simulink model "full_R2016b"  (R2017a)
settings: Solver=VariableStepAuto  StartTime=0.0  StopTime=10.0  RelTol=1e-3
libraries: aerolibconvert2 x2, aerolibgravity2 x2
settings Model: Creator=decla  LastModifiedBy=decla
settings DataIOCC: ReturnWorkspaceOutputs=on
settings SFSimCC: SimUseLocalCustomCode=on
settings RTWCC: RTWUseLocalCustomCode=on

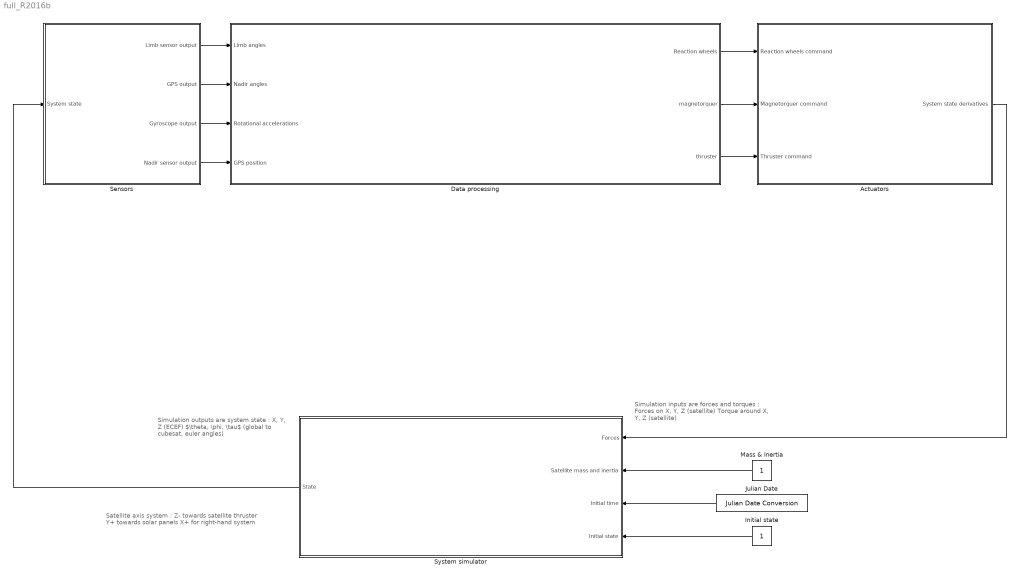
== system full_R2016b ==
  note: Simulation outputs are system state :
      | X, Y, Z (ECEF)
      | $\theta, \phi, \tau$ (global to cubesat, euler angles)
  note: Simulation inputs are forces and torques :
      | Forces on X, Y, Z (satellite)
      | Torque around X, Y, Z (satellite)
  note: Satellite axis system :
      | Z- towards satellite thruster
      | Y+ towards solar panels
      | X+ for right-hand system
  Actuators : Subsystem
  Data processing : Subsystem
  Initial state : Constant
  Julian Date : aerolibconvert2/Julian Date Conversion  year=2004  month=October  day=10  hour=12  min=21  sec=0  modflag=off  deltaT=None  errorflag=Error
      settings: SourceProductBaseCode=AE
  Mass & Inertia : Constant
  Sensors : Subsystem
  System simulator : Subsystem
  wires:
  Data processing/3(thruster) -> Actuators/3(Thruster command)
  Actuators/1(System state derivatives) -> System simulator/1(Forces)
  System simulator/1(State) -> Sensors/1(System state)
  Sensors/4(Nadir sensor output) -> Data processing/4(GPS position)
  Sensors/3(Gyroscope output) -> Data processing/3(Rotational accelerations)
  Sensors/2(GPS output) -> Data processing/2(Nadir angles)
  Sensors/1(Limb sensor output) -> Data processing/1(Limb angles)
  Data processing/2(magnetorquer) -> Actuators/2(Magnetorquer command)
  Data processing/1(Reaction wheels) -> Actuators/1(Reaction wheels command)
  Mass & Inertia/1 -> System simulator/2(Satellite mass and inertia)
  Julian Date/1 -> System simulator/3(Initial time)
  Initial state/1 -> System simulator/4(Initial state)

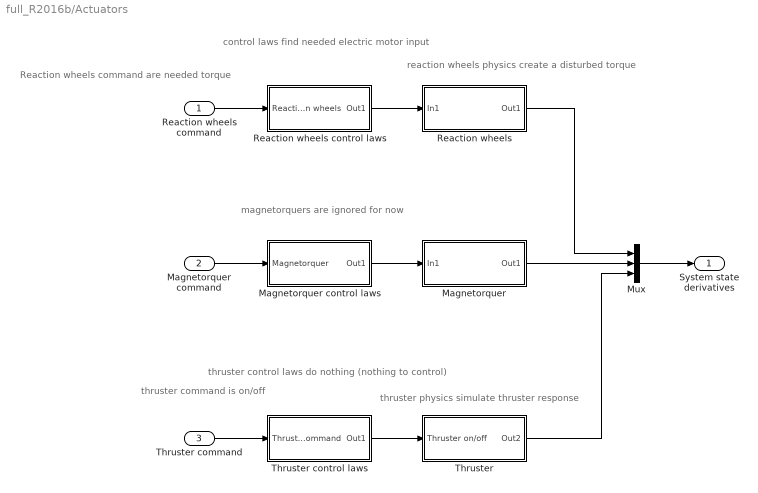
== system full_R2016b/Actuators ==
  note: magnetorquers are ignored for now
  note: thruster control laws do nothing (nothing to control)
  note: thruster physics simulate thruster response
  note: thruster command is on/off
  note: reaction wheels physics create a disturbed torque
  note: control laws find needed electric motor input
  note: Reaction wheels command are needed torque
  Reaction wheels command : Inport
  Magnetorquer command : Inport  Port=2
  Thruster command : Inport  Port=3
  Magnetorquer : Subsystem
  Magnetorquer control laws : Subsystem
  Mux : Mux  Inputs=3
  Reaction wheels : Subsystem
  Reaction wheels control laws : Subsystem
  Thruster : Subsystem
  Thruster control laws : Subsystem
  System state derivatives : Outport
  wires:
  Reaction wheels command/1 -> Reaction wheels control laws/1(Reaction wheels)
  Magnetorquer command/1 -> Magnetorquer control laws/1(Magnetorquer)
  Thruster command/1 -> Thruster control laws/1(Thruster command)
  Thruster control laws/1(Out1) -> Thruster/1(Thruster on/off)
  Magnetorquer control laws/1(Out1) -> Magnetorquer/1(In1)
  Reaction wheels control laws/1(Out1) -> Reaction wheels/1(In1)
  Thruster/1(Out2) -> Mux/3
  Magnetorquer/1(Out1) -> Mux/2
  Reaction wheels/1(Out1) -> Mux/1
  Mux/1 -> System state derivatives/1

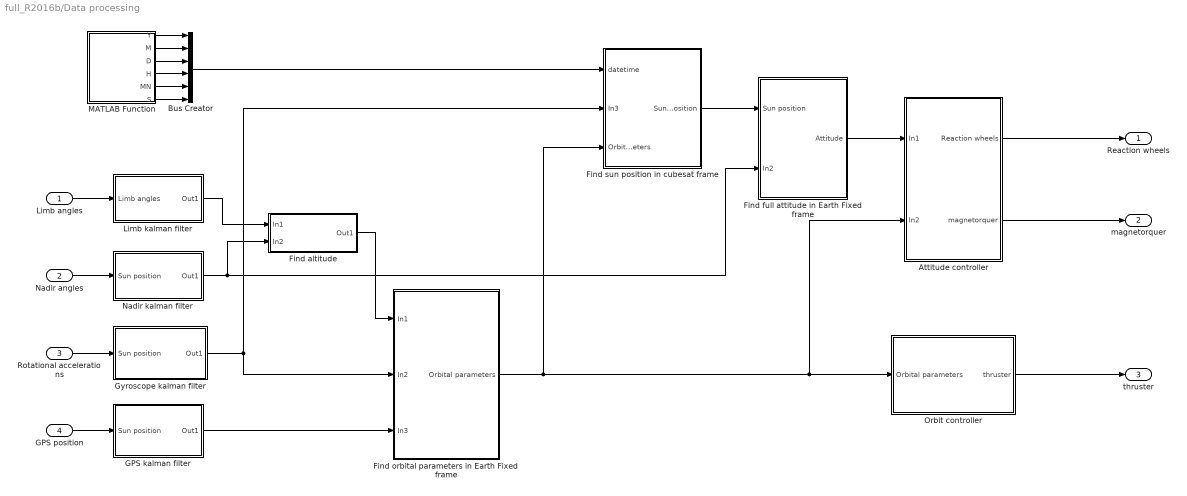
== system full_R2016b/Data processing ==
  Limb angles : Inport
  Nadir angles : Inport  Port=2
  Rotational accelerations : Inport  Port=3
  GPS position : Inport  Port=4
  Attitude controller : Subsystem
  Bus Creator : BusCreator  Inputs=6
  Find altitude : Subsystem
  Find full attitude in Earth Fixed frame : Subsystem
  Find orbital parameters in Earth Fixed frame : Subsystem
  Find sun position in cubesat frame : Subsystem
  GPS kalman filter : Subsystem
  Gyroscope kalman filter : Subsystem
  Limb kalman filter : Subsystem
  MATLAB Function : MATLAB Function  TreatAsAtomicUnit=on
  Nadir kalman filter : Subsystem
  Orbit controller : Subsystem
  Reaction wheels : Outport
  magnetorquer : Outport  Port=2
  thruster : Outport  Port=3
  wires:
  Limb angles/1 -> Limb kalman filter/1(Limb angles)
  Nadir angles/1 -> Nadir kalman filter/1(Sun position)
  Rotational accelerations/1 -> Gyroscope kalman filter/1(Sun position)
  GPS position/1 -> GPS kalman filter/1(Sun position)
  Gyroscope kalman filter/1(Out1) -> Find orbital parameters in Earth Fixed frame/2(In2), Find sun position in cubesat frame/2(In3)
  GPS kalman filter/1(Out1) -> Find orbital parameters in Earth Fixed frame/3(In3)
  Find sun position in cubesat frame/1(Sun position) -> Find full attitude in Earth Fixed frame/1(Sun position)
  Find orbital parameters in Earth Fixed frame/1(Orbital parameters) -> Find sun position in cubesat frame/3(Orbital parameters), Orbit controller/1(Orbital parameters), Attitude controller/2(In2)
  Orbit controller/1(thruster) -> thruster/1
  Attitude controller/1(Reaction wheels) -> Reaction wheels/1
  Attitude controller/2(magnetorquer) -> magnetorquer/1
  Find full attitude in Earth Fixed frame/1(Attitude) -> Attitude controller/1(In1)
  MATLAB Function/1(Y) -> Bus Creator/1
  MATLAB Function/2(M) -> Bus Creator/2
  MATLAB Function/3(D) -> Bus Creator/3
  MATLAB Function/4(H) -> Bus Creator/4
  MATLAB Function/5(MN) -> Bus Creator/5
  MATLAB Function/6(S) -> Bus Creator/6
  Bus Creator/1 -> Find sun position in cubesat frame/1(datetime)
  Limb kalman filter/1(Out1) -> Find altitude/1(In1)
  Nadir kalman filter/1(Out1) -> Find full attitude in Earth Fixed frame/2(In2), Find altitude/2(In2)
  Find altitude/1(Out1) -> Find orbital parameters in Earth Fixed frame/1(In1)

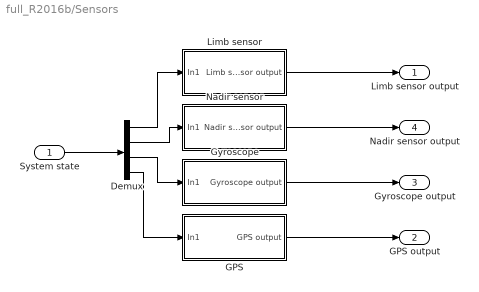
== system full_R2016b/Sensors ==
  System state : Inport
  Demux : Demux
  GPS : Subsystem
  Gyroscope : Subsystem
  Limb sensor : Subsystem
  Nadir sensor : Subsystem
  Limb sensor output : Outport
  GPS output : Outport  Port=2
  Gyroscope output : Outport  Port=3
  Nadir sensor output : Outport  Port=4
  wires:
  Demux/4 -> GPS/1(In1)
  Demux/3 -> Gyroscope/1(In1)
  Nadir sensor/1(Nadir sensor output) -> Nadir sensor output/1
  Limb sensor/1("Limb sensor output ") -> Limb sensor output/1
  Gyroscope/1(Gyroscope output) -> Gyroscope output/1
  GPS/1(GPS output) -> GPS output/1
  Demux/2 -> Nadir sensor/1(In1)
  System state/1 -> Demux/1
  Demux/1 -> Limb sensor/1(In1)

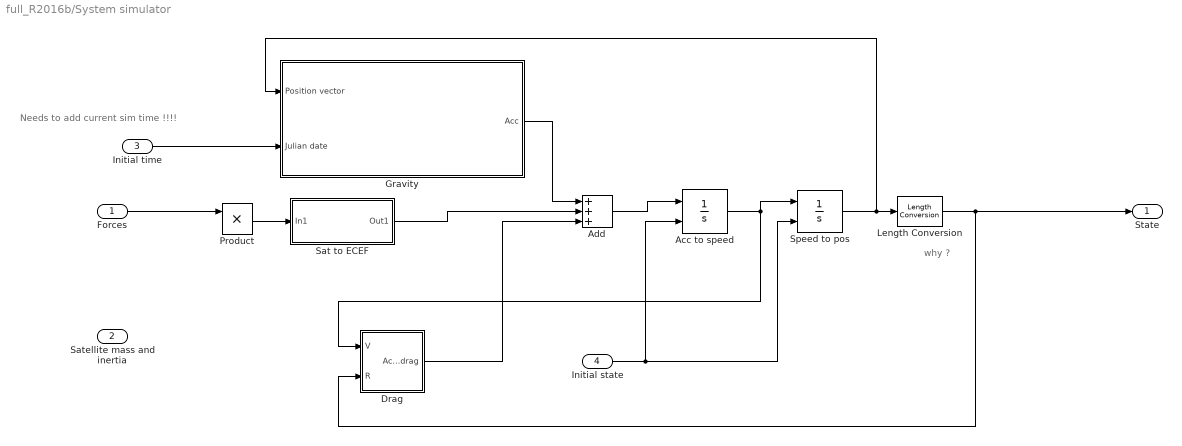
== system full_R2016b/System simulator ==
  note: why ?
  note: Needs to add current sim time !!!!
  Forces : Inport
  Satellite mass and inertia : Inport  Port=2
  Initial time : Inport  Port=3
  Initial state : Inport  Port=4
  Acc to speed : Integrator  InitialConditionSource=external  InitialCondition=[-2871.828;-5954.63;3774.64]
  Add : Sum  Inputs=+++
  Drag : Subsystem
  Gravity : Subsystem
  Length Conversion : aerolibconvert2/Length Conversion  IU=m  OU=km
  Product : Product
  Sat to ECEF : Subsystem
  Speed to pos : Integrator  InitialConditionSource=external  InitialCondition=[2383.89e3;2594.67e3;5906.12e3]
  State : Outport
  wires:
  Drag/1(Acc_drag) -> Add/3
  Add/1 -> Acc to speed/1
  Gravity/1(Acc) -> Add/1
  Speed to pos/1 -> Length Conversion/1, Gravity/1(Position vector)
  Acc to speed/1 -> Drag/1(V), Speed to pos/1
  Length Conversion/1 -> State/1, Drag/2(R)
  Sat to ECEF/1(Out1) -> Add/2
  Forces/1 -> Product/1
  Product/1 -> Sat to ECEF/1(In1)
  Initial time/1 -> Gravity/2(Julian date)
  Initial state/1 -> Speed to pos/2, Acc to speed/2

== system full_R2016b/Actuators/Magnetorquer ==
  In1 : Inport
  Out1 : Outport
  wires:
  In1/1 -> Out1/1

== system full_R2016b/Actuators/Magnetorquer control laws ==
  Magnetorquer : Inport
  Out1 : Outport
  wires:
  Magnetorquer/1 -> Out1/1

== system full_R2016b/Actuators/Reaction wheels ==
  In1 : Inport
  Out1 : Outport
  wires:
  In1/1 -> Out1/1

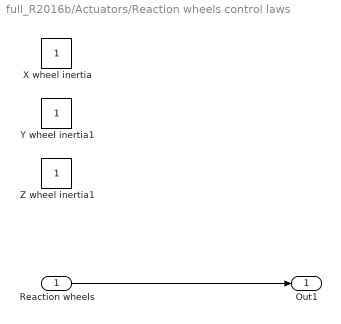
== system full_R2016b/Actuators/Reaction wheels control laws ==
  Reaction wheels : Inport
  X wheel inertia : Constant
  Y wheel inertia1 : Constant
  Z wheel inertia1 : Constant
  Out1 : Outport
  wires:
  Reaction wheels/1 -> Out1/1

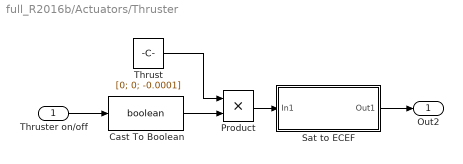
== system full_R2016b/Actuators/Thruster ==
  Thruster on/off : Inport
  Cast To Boolean : DataTypeConversion  OutDataTypeStr=boolean
  Product : Product
  Sat to ECEF : Subsystem
  Thrust : Constant  Value=[0; 0; -0.0001]
  Out2 : Outport
  wires:
  Product/1 -> Sat to ECEF/1(In1)
  Thrust/1 -> Product/1
  Thruster on/off/1 -> Cast To Boolean/1
  Sat to ECEF/1(Out1) -> Out2/1
  Cast To Boolean/1 -> Product/2

== system full_R2016b/Actuators/Thruster control laws ==
  Thruster command : Inport
  Out1 : Outport
  wires:
  Thruster command/1 -> Out1/1

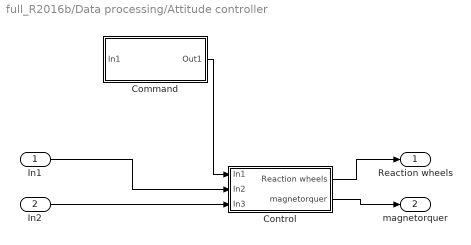
== system full_R2016b/Data processing/Attitude controller ==
  In1 : Inport
  In2 : Inport  Port=2
  Command : Subsystem
  Control : Subsystem
  Reaction wheels : Outport
  magnetorquer : Outport  Port=2
  wires:
  In2/1 -> Control/3(In3)
  In1/1 -> Control/2(In2)
  Control/2(magnetorquer) -> magnetorquer/1
  Control/1(Reaction wheels) -> Reaction wheels/1
  Command/1(Out1) -> Control/1(In1)

== system full_R2016b/Data processing/Find altitude ==
  In1 : Inport
  In2 : Inport  Port=2
  Out1 : Outport
  wires:
  In1/1 -> Out1/1

== system full_R2016b/Data processing/Find full attitude in Earth Fixed frame ==
  Sun position : Inport
  In2 : Inport  Port=2
  Attitude : Outport
  wires:
  Sun position/1 -> Attitude/1

== system full_R2016b/Data processing/Find orbital parameters in Earth Fixed frame ==
  In1 : Inport
  In2 : Inport  Port=2
  In3 : Inport  Port=3
  Orbital parameters : Outport
  wires:
  In1/1 -> Orbital parameters/1

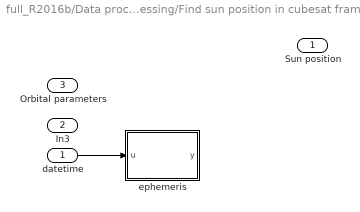
== system full_R2016b/Data processing/Find sun position in cubesat frame ==
  datetime : Inport
  In3 : Inport  Port=2
  Orbital parameters : Inport  Port=3
  ephemeris : MATLAB Function  TreatAsAtomicUnit=on
  Sun position : Outport
  wires:
  ? -> Sun position/1
  datetime/1 -> ephemeris/1(u)

== system full_R2016b/Data processing/GPS kalman filter ==
  Sun position : Inport
  Out1 : Outport
  wires:
  Sun position/1 -> Out1/1

== system full_R2016b/Data processing/Gyroscope kalman filter ==
  Sun position : Inport
  Out1 : Outport
  wires:
  Sun position/1 -> Out1/1

== system full_R2016b/Data processing/Limb kalman filter ==
  Limb angles : Inport
  Out1 : Outport
  wires:
  Limb angles/1 -> Out1/1

== system full_R2016b/Data processing/Nadir kalman filter ==
  Sun position : Inport
  Out1 : Outport
  wires:
  Sun position/1 -> Out1/1

== system full_R2016b/Data processing/Orbit controller ==
  Orbital parameters : Inport
  Command : Subsystem
  Control : Subsystem
  thruster : Outport
  wires:
  Command/1(Out1) -> Control/2(In1)
  Orbital parameters/1 -> Control/1(Orbital parameters)
  Control/1(Out1) -> thruster/1

== system full_R2016b/Sensors/GPS ==
  In1 : Inport
  MATLAB Function : MATLAB Function  TreatAsAtomicUnit=on
  GPS output : Outport
  wires:
  In1/1 -> MATLAB Function/1(SystemStates)
  MATLAB Function/1(GPS_position) -> GPS output/1

== system full_R2016b/Sensors/Gyroscope ==
  In1 : Inport
  Derivative : Derivative
  Derivative1 : Derivative
  Gyroscope output : Outport
  wires:
  In1/1 -> Derivative/1
  Derivative/1 -> Derivative1/1
  Derivative1/1 -> Gyroscope output/1

== system full_R2016b/Sensors/Limb sensor ==
  In1 : Inport
  MATLAB Function : MATLAB Function  TreatAsAtomicUnit=on
  "Limb sensor output " : Outport
  wires:
  In1/1 -> MATLAB Function/1(SystemStates)
  MATLAB Function/1(LimbAngle) -> "Limb sensor output "/1

== system full_R2016b/Sensors/Nadir sensor ==
  In1 : Inport
  MATLAB Function : MATLAB Function  TreatAsAtomicUnit=on
  Nadir sensor output : Outport
  wires:
  In1/1 -> MATLAB Function/1(SystemStates)
  MATLAB Function/1(NadirAngle) -> Nadir sensor output/1

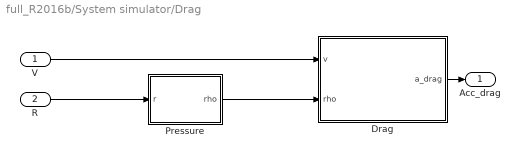
== system full_R2016b/System simulator/Drag ==
  V : Inport
  R : Inport  Port=2
  Drag : MATLAB Function  TreatAsAtomicUnit=on
  Pressure : MATLAB Function  TreatAsAtomicUnit=on
  Acc_drag : Outport
  wires:
  Pressure/1(rho) -> Drag/2(rho)
  Drag/1(a_drag) -> Acc_drag/1
  V/1 -> Drag/1(v)
  R/1 -> Pressure/1(r)

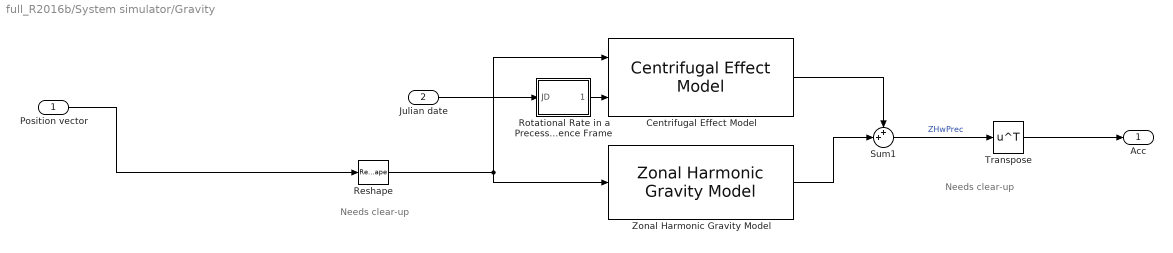
== system full_R2016b/System simulator/Gravity ==
  note: Needs clear-up
  note: Needs clear-up
  Position vector : Inport
  Julian date : Inport  Port=2
  Centrifugal Effect Model : aerolibgravity2/Centrifugal Effect Model  ptype=Custom  omega=7.2921150e-005  rate_loc=on
      settings: SourceProductBaseCode=AE
  Reshape : Reshape  OutputDimensionality=Row vector (2-D)
  Rotational Rate in a Precessing Reference Frame : Subsystem
  Sum1 : Sum  Inputs=++|
  Transpose : Math  Operator=transpose  SaturateOnIntegerOverflow=on
  Zonal Harmonic Gravity Model : aerolibgravity2/Zonal Harmonic Gravity Model  units=Metric (MKS)  degree=4  action=Warning  ptype=Earth  R=6378136.3  GM=398600441500000  jvalue=[1.0826269e-03 -2.5323000e-06 -1.6204000e-06]
      settings: SourceProductBaseCode=AE
  Acc : Outport
  wires:
  Reshape/1 -> Centrifugal Effect Model/1, Zonal Harmonic Gravity Model/1
  Rotational Rate in a Precessing Reference Frame/1(omega) -> Centrifugal Effect Model/2
  Position vector/1 -> Reshape/1
  Julian date/1 -> Rotational Rate in a Precessing Reference Frame/1(JD)
  Zonal Harmonic Gravity Model/1 -> Sum1/2
  Centrifugal Effect Model/1 -> Sum1/1
  Sum1/1 -> Transpose/1  "ZHwPrec"
  Transpose/1 -> Acc/1

== system full_R2016b/System simulator/Sat to ECEF ==
  In1 : Inport
  Out1 : Outport
  wires:
  In1/1 -> Out1/1

== system full_R2016b/Actuators/Thruster/Sat to ECEF ==
  In1 : Inport
  Out1 : Outport
  wires:
  In1/1 -> Out1/1

== system full_R2016b/Data processing/Attitude controller/Command ==
  In1 : Inport
  Out1 : Outport
  wires:
  In1/1 -> Out1/1

== system full_R2016b/Data processing/Attitude controller/Control ==
  In1 : Inport
  In2 : Inport  Port=2
  In3 : Inport  Port=3
  Reaction wheels : Outport
  magnetorquer : Outport  Port=2
  wires:
  In1/1 -> Reaction wheels/1

== system full_R2016b/Data processing/Orbit controller/Command ==
  In1 : Inport
  Constant : Constant
  Out1 : Outport
  wires:
  In1/1 -> Out1/1

== system full_R2016b/Data processing/Orbit controller/Control ==
  Orbital parameters : Inport
  In1 : Inport  Port=2
  Out1 : Outport
  wires:
  Orbital parameters/1 -> Out1/1

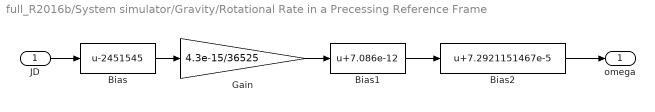
== system full_R2016b/System simulator/Gravity/Rotational Rate in a Precessing Reference Frame ==
  JD : Inport
  Bias : Bias  Bias=-2451545
  Bias1 : Bias  Bias=7.086e-12
  Bias2 : Bias  Bias=7.2921151467e-5
  Gain : Gain  Gain=4.3e-15/36525
  omega : Outport
  wires:
  JD/1 -> Bias/1
  Bias/1 -> Gain/1
  Gain/1 -> Bias1/1
  Bias1/1 -> Bias2/1
  Bias2/1 -> omega/1

== matlab function full_R2016b/Data processing/Find sun position in cubesat frame/ephemeris ==
  data: u input; y output
% https://ssd.jpl.nasa.gov/?planet_pos
function y = fcn(u)

y = u;

== matlab function full_R2016b/Data processing/MATLAB Function ==
  data: Y output; M output; D output; H output; MN output; S output
% https://www.mathworks.com/matlabcentral/answers/30479-how-to-get-system-date-and-time-into-simulink
function [Y, M, D, H, MN, S] = sysClock()
   coder.extrinsic('clock');
   Y = 0;
   M = 0;
   D = 0;
   H = 0;
   MN = 0;
   S = 0;
   [Y, M, D, H, MN, S] = clock;
end

== matlab function full_R2016b/System simulator/Drag/Drag ==
  data: v input; a_drag output; rho input
function a_drag = fcn(v, rho)
area = 100e-4;
mass = 3;
V = norm(v);
Cd = 1.05;

a_drag = -0.5*Cd*(area/mass)*rho*V^2;

== matlab function full_R2016b/System simulator/Drag/Pressure ==
  data: r input; rho output
function rho = fcn(r)
alt = norm(r);
A = 1.140564e-10;
B = -2.130756e-7;
C = 1.570562e-4;
D = -0.07029296;
E = -12.89844;

rho = exp(A*alt^4 + B*alt^3 + C*alt^2 + D*alt + E);

== matlab function full_R2016b/Sensors/GPS/MATLAB Function ==
  data: SystemStates input; GPS_position output
function GPS_position   = GPS_function(SystemStates)
% En faisant l'hypothèse que SystemStates = ([rotX rotY rotZ],[X Y Z])

noise_pos = 0 + (10-0) .* rand(1,1) % bruit pour la position
%noise_speed = 0 + (0.25-0) .* rand(1,1) % bruit pour la vitesse
GPS_position = SystemStates(2) + noise_pos

end

== matlab function full_R2016b/Sensors/Limb sensor/MATLAB Function ==
  data: SystemStates input; LimbAngle output
function LimbAngle   = Limb_function( SystemStates )
% En faisant l'hypothèse que SystemStates = ([rotX rotY rotZ],[X Y Z])
noise = 0 + (0.25-0) .* rand(1,1)
position = SystemStates(2)

NadirAngle = -position + noise + acrtan(6371/ sqrt(position(1)^2 + position(2)^2 + position(3)^2)) 

end

== matlab function full_R2016b/Sensors/Nadir sensor/MATLAB Function ==
  data: SystemStates input; NadirAngle output
function NadirAngle   = Nadir_function(SystemStates)
% En faisant l'hypothèse que SystemStates = ([rotX rotY rotZ],[X Y Z])
noise = 0 + (0.25-0) .* rand(1,1)
position = SystemStates(2)
NadirAngle = -position + noise
end
